simulink model "chap6_1sim"  (R2015a)
settings: Solver=ode45  StartTime=0.0  StopTime=10  FixedStep=0.01  RelTol=1e-3
settings Model: Creator=Masoud  LastModifiedBy=Masoud

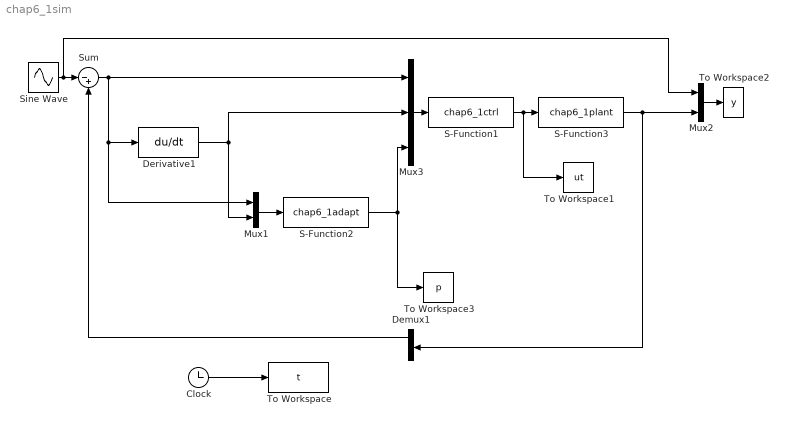
== system chap6_1sim ==
  Clock : Clock
  Demux1 : Demux  Outputs=2
  Derivative1 : Derivative
  Mux1 : Mux  Inputs=2
  Mux2 : Mux  Inputs=2
  Mux3 : Mux  Inputs=3
  S-Function1 : S-Function  FunctionName=chap6_1ctrl  SFunctionModules='chap6_1ctrl'
  S-Function2 : S-Function  FunctionName=chap6_1adapt  SFunctionModules='chap6_1adapt'
  S-Function3 : S-Function  FunctionName=chap6_1plant  SFunctionModules='chap6_1plant'
  Sine Wave : Sin  Frequency=0.3*pi  SampleTime=0
  Sum : Sum  Inputs=|-+
  To Workspace : ToWorkspace  VariableName=t  SampleTime=-1
  To Workspace1 : ToWorkspace  VariableName=ut  SampleTime=-1
  To Workspace2 : ToWorkspace  VariableName=y  SampleTime=-1
  To Workspace3 : ToWorkspace  VariableName=p  SampleTime=-1
  wires:
  Clock/1 -> To Workspace/1
  Mux1/1 -> S-Function2/1
  Mux2/1 -> To Workspace2/1
  S-Function3/1 -> Mux2/2, Demux1/1
  S-Function2/1 -> To Workspace3/1, Mux3/3
  S-Function1/1 -> S-Function3/1, To Workspace1/1
  Derivative1/1 -> Mux1/2, Mux3/2
  Sine Wave/1 -> Mux2/1, Sum/1
  Sum/1 -> Mux1/1, Derivative1/1, Mux3/1
  Demux1/1 -> Sum/2
  Mux3/1 -> S-Function1/1
